simulink model "satellite"  (R2018a)
settings: Solver=VariableStepAuto  StartTime=0.0  StopTime=20  RelTol=1e-3
libraries: sharedutil x2
settings Model: Creator=Siddharth Deore  LastModifiedBy=Siddharth Deore

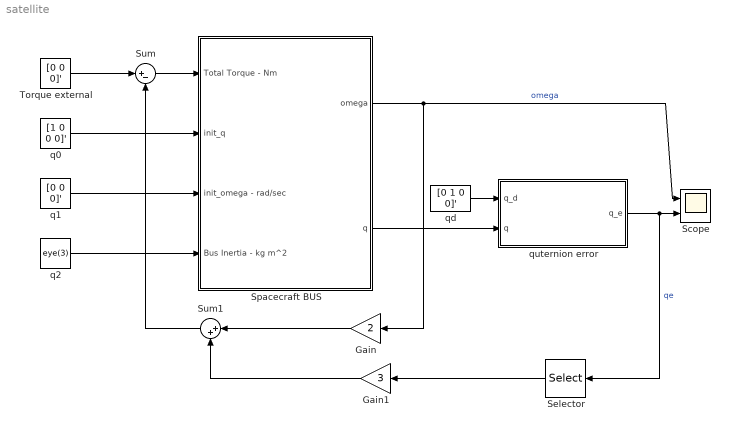
== system satellite ==
  Gain : Gain  Gain=2
  Gain1 : Gain  Gain=3
  Scope : Scope  NumInputPorts=2
  Selector : Selector  InputPortWidth=4  IndexOptions=Index vector (dialog)  Indices=[1 2 3 ]  OutputSizes=1
  Spacecraft BUS : Subsystem
  Sum : Sum  Inputs=|+-
  Sum1 : Sum  Inputs=|++
  Torque external : Constant  Value=[0 0 0]'
  q0 : Constant  Value=[1 0 0 0]'
  q1 : Constant  Value=[0 0 0]'
  q2 : Constant  Value=eye(3)
  qd : Constant  Value=[0 1 0 0]'
  quternion error : Subsystem
  wires:
  q0/1 -> Spacecraft BUS/2(init_q)
  q1/1 -> Spacecraft BUS/3(init_omega - rad/sec)
  q2/1 -> Spacecraft BUS/4(Bus Inertia - kg m^2)
  Spacecraft BUS/1(omega) -> Gain/1, Scope/1  "omega"
  Spacecraft BUS/2(q) -> quternion error/2(q)
  qd/1 -> quternion error/1(q_d)
  Torque external/1 -> Sum/1
  Sum/1 -> Spacecraft BUS/1(Total Torque - Nm)
  quternion error/1(q_e) -> Selector/1, Scope/2  "qe"
  Selector/1 -> Gain1/1
  Gain/1 -> Sum1/1
  Gain1/1 -> Sum1/2
  Sum1/1 -> Sum/2

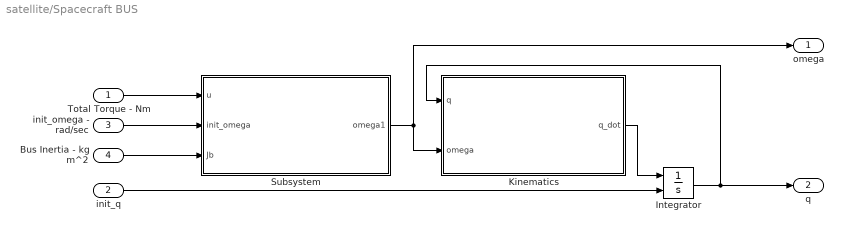
== system satellite/Spacecraft BUS ==
  Total Torque - Nm : Inport
  init_q : Inport  Port=2
  init_omega - rad/sec : Inport  Port=3
  Bus Inertia - kg m^2 : Inport  Port=4
  Integrator : Integrator  InitialConditionSource=external
  Kinematics : Subsystem
  Subsystem : Subsystem
  omega : Outport
  q : Outport  Port=2
  wires:
  Kinematics/1(q_dot) -> Integrator/1
  Integrator/1 -> Kinematics/1(q), q/1
  Total Torque - Nm/1 -> Subsystem/1(u)
  init_omega - rad/sec/1 -> Subsystem/2(init_omega)
  init_q/1 -> Integrator/2
  Subsystem/1(omega1) -> Kinematics/2(omega), omega/1
  Bus Inertia - kg m^2/1 -> Subsystem/3(Jb)

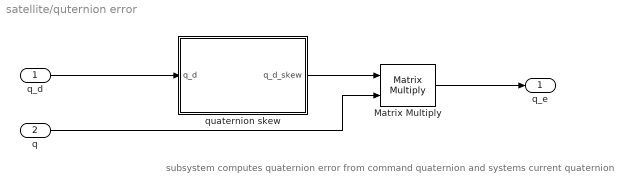
== system satellite/quternion error ==
  note: subsystem computes quaternion error from command quaternion and systems current quaternion
  q_d : Inport
  q : Inport  Port=2
  Matrix Multiply : Product  Multiplication=Matrix(*)
  quaternion skew : Subsystem
  q_e : Outport
  wires:
  quaternion skew/1(q_d_skew) -> Matrix Multiply/1
  Matrix Multiply/1 -> q_e/1
  q/1 -> Matrix Multiply/2
  q_d/1 -> quaternion skew/1(q_d)

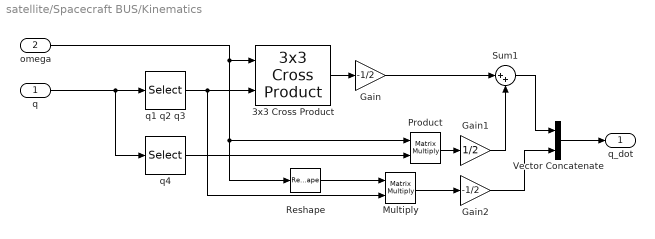
== system satellite/Spacecraft BUS/Kinematics ==
  q : Inport
  omega : Inport  Port=2
  3x3 Cross Product : sharedutil/3x3 Cross Product  aMode=aMode
      settings: SourceProductBaseCode=AE
  Gain : Gain  Gain=-1/2
  Gain1 : Gain  Gain=1/2
  Gain2 : Gain  Gain=-1/2
  Multiply : Product  Multiplication=Matrix(*)
  Product : Product  Multiplication=Matrix(*)
  Reshape : Reshape  OutputDimensionality=Row vector (2-D)
  Sum1 : Sum  Inputs=|++
  Vector Concatenate : Concatenate
  q1 q2 q3 : Selector  InputPortWidth=4  IndexOptions=Index vector (dialog)  Indices=[1 2 3]  OutputSizes=1
  q4 : Selector  InputPortWidth=4  IndexOptions=Index vector (dialog)  Indices=[4]  OutputSizes=1
  q_dot : Outport
  wires:
  omega/1 -> 3x3 Cross Product/1, Product/1, Reshape/1
  q/1 -> q4/1, q1 q2 q3/1
  q1 q2 q3/1 -> Multiply/2, 3x3 Cross Product/2
  Gain1/1 -> Sum1/2
  3x3 Cross Product/1 -> Gain/1
  Product/1 -> Gain1/1
  Multiply/1 -> Gain2/1
  Gain/1 -> Sum1/1
  q4/1 -> Product/2
  Sum1/1 -> Vector Concatenate/1
  Gain2/1 -> Vector Concatenate/2
  Reshape/1 -> Multiply/1
  Vector Concatenate/1 -> q_dot/1

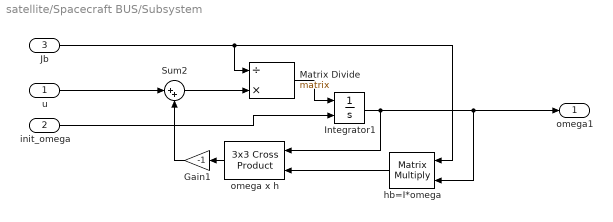
== system satellite/Spacecraft BUS/Subsystem ==
  u : Inport
  init_omega : Inport  Port=2
  Jb : Inport  Port=3
  Gain1 : Gain  Gain=-1
  Integrator1 : Integrator  InitialConditionSource=external  ZeroCross=off
  Matrix Divide : Product  Inputs=/*  Multiplication=Matrix(*)
  Sum2 : Sum  Inputs=|++
  hb=I*omega : Product  Multiplication=Matrix(*)
  omega x h : sharedutil/3x3 Cross Product  aMode=aMode
      settings: SourceProductBaseCode=AE
  omega1 : Outport
  wires:
  Gain1/1 -> Sum2/2
  Integrator1/1 -> omega x h/1, omega1/1, hb=I*omega/2
  init_omega/1 -> Integrator1/2
  Sum2/1 -> Matrix Divide/2
  hb=I*omega/1 -> omega x h/2
  omega x h/1 -> Gain1/1
  u/1 -> Sum2/1
  Matrix Divide/1 -> Integrator1/1
  Jb/1 -> Matrix Divide/1, hb=I*omega/1

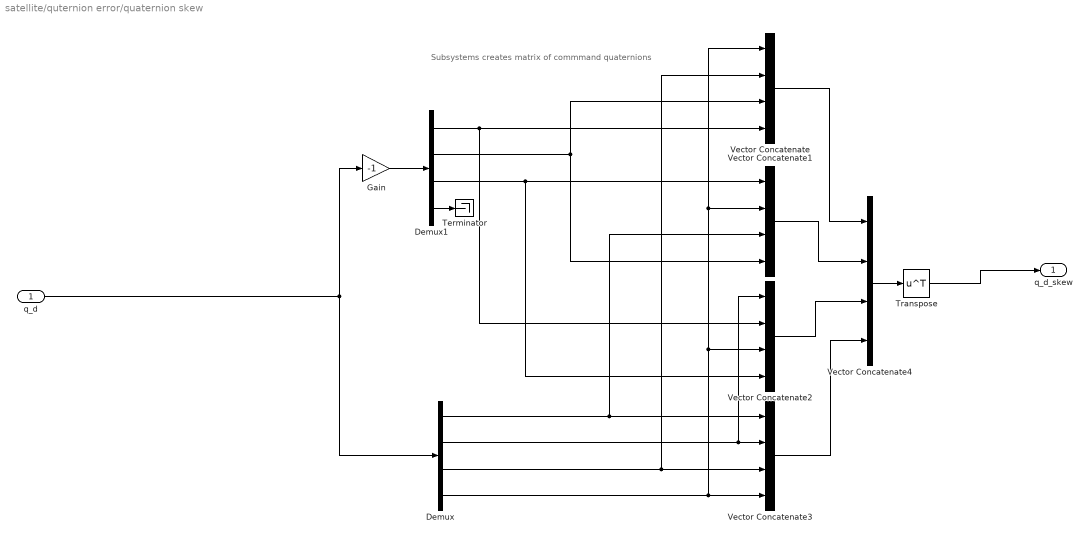
== system satellite/quternion error/quaternion skew ==
  note: Subsystems creates matrix of commmand quaternions
  q_d : Inport
  Demux : Demux
  Demux1 : Demux
  Gain : Gain  Gain=-1
  Terminator : Terminator
  Transpose : Math  Operator=transpose  SaturateOnIntegerOverflow=on
  Vector Concatenate{,1..3} (4 alike) : Concatenate  NumInputs=4
  Vector Concatenate4 : Concatenate  NumInputs=4  Mode=Multidimensional array  ConcatenateDimension=[2]
  q_d_skew : Outport
  wires:
  Demux1/3 -> Vector Concatenate2/4, Vector Concatenate1/1
  q_d/1 -> Gain/1, Demux/1
  Demux/1 -> Vector Concatenate1/3, Vector Concatenate3/1
  Demux/4 -> Vector Concatenate/1, Vector Concatenate1/2, Vector Concatenate2/3, Vector Concatenate3/4
  Vector Concatenate3/1 -> Vector Concatenate4/4
  Demux1/2 -> Vector Concatenate1/4, Vector Concatenate/3
  Demux1/1 -> Vector Concatenate2/2, Vector Concatenate/4
  Demux/2 -> Vector Concatenate3/2, Vector Concatenate2/1
  Vector Concatenate4/1 -> Transpose/1
  Gain/1 -> Demux1/1
  Demux/3 -> Vector Concatenate/2, Vector Concatenate3/3
  Vector Concatenate2/1 -> Vector Concatenate4/3
  Vector Concatenate1/1 -> Vector Concatenate4/2
  Demux1/4 -> Terminator/1
  Vector Concatenate/1 -> Vector Concatenate4/1
  Transpose/1 -> q_d_skew/1
